simulink model "Slip_Calculation_TestHarness"  (R2023b)
settings: Solver=FixedStepDiscrete  StartTime=0.01  StopTime=12.0  RelTol=1e-3
libraries: simulink x1, SignalEditorBlockLib x1
settings Model: Creator=E8KUAVE  LastModifiedBy=E8KUAVE

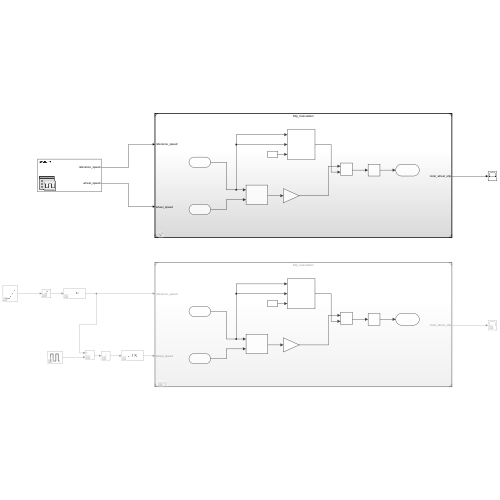
[thumbnail: Simulink's stored preview of the top-level diagram]
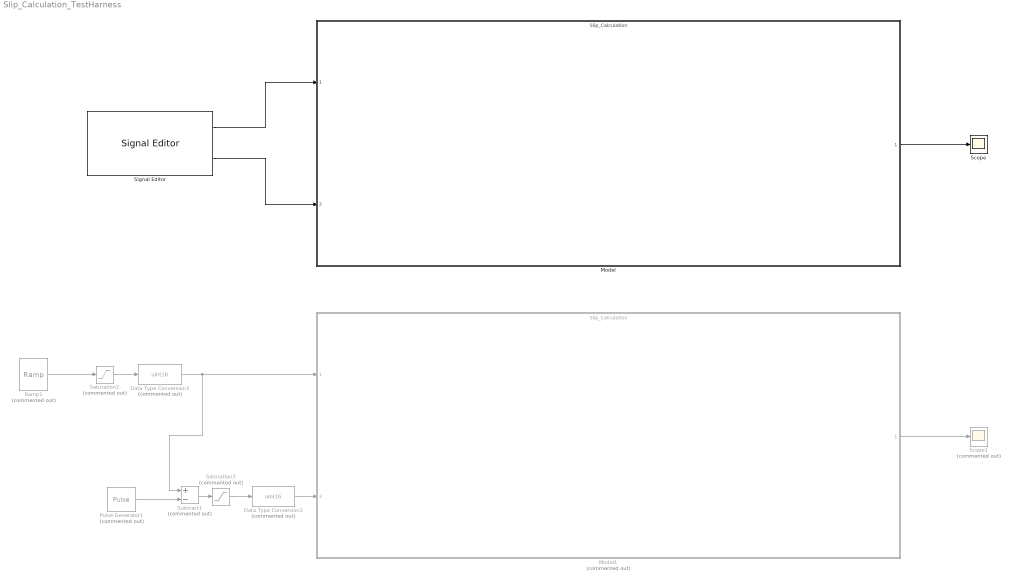
== system Slip_Calculation_TestHarness ==
  Data Type Conversion2 : DataTypeConversion  Commented=on  OutDataTypeStr=uint16  SaturateOnIntegerOverflow=off  RndMeth=Floor
  Data Type Conversion3 : DataTypeConversion  Commented=on  OutDataTypeStr=uint16  SaturateOnIntegerOverflow=off  RndMeth=Floor
  Model : ModelReference  ModelNameDialog=Slip_Calculation.slx  SimulationMode=Normal  ModelReferenceVersion=1.3
  Model1 : ModelReference  Commented=on  ModelNameDialog=Slip_Calculation.slx  SimulationMode=Normal  ModelReferenceVersion=1.3
  Pulse Generator1 : DiscretePulseGenerator  Commented=on  PulseType=Time based  Amplitude=40  Period=10  PulseWidth=20  PhaseDelay=3
  Ramp1 : simulink/Sources/Ramp  Commented=on  slope=-15  start=0  InitialOutput=150
  Saturation2 : Saturate  Commented=on  UpperLimit=150  LowerLimit=0
  Saturation3 : Saturate  Commented=on  UpperLimit=150  LowerLimit=0
  Scope : Scope
  Scope1 : Scope  Commented=on
  Signal Editor : SignalEditorBlockLib/Signal Editor  FileName=C:\Users\E8KUAVE\Documents\Work\Coding\Platform_Neutral_FreeRTOS\MATLAB_ApplicationCode\Tests\sign_editor_test.mat  ActiveScenario=Scenario  ActiveSignal=reference_speed  IsBus=off  OutputBusObjectStr=Bus: BusObject  SampleTime=0  Interpolate=off  ZeroCross=off  OutputAfterFinalValue=Setting to zero  Unit=inherit  PreserveSignalName=on  ApplySigPropsToAllScenarios=on  ApplySigPropsToAllSignals=off
  Subtract1 : Sum  Commented=on  Inputs=+-  OutDataTypeStr=uint16
  wires:
  Model/1 -> Scope/1
  Data Type Conversion3/1 -> Subtract1/1, Model1/1
  Model1/1 -> Scope1/1
  Saturation3/1 -> Data Type Conversion2/1
  Saturation2/1 -> Data Type Conversion3/1
  Subtract1/1 -> Saturation3/1
  Pulse Generator1/1 -> Subtract1/2
  Data Type Conversion2/1 -> Model1/2
  Ramp1/1 -> Saturation2/1
  Signal Editor/1 -> Model/1
  Signal Editor/2 -> Model/2
